simulink model "train_model"  (R2024b)
settings: Solver=VariableStepAuto  StartTime=0.0  StopTime=10.0  RelTol=1e-3
InitFcn:
  | m = 10000;
libraries: fuzblock x1
settings Model: Creator=Jan Tepel  LastModifiedBy=Jan Tepel

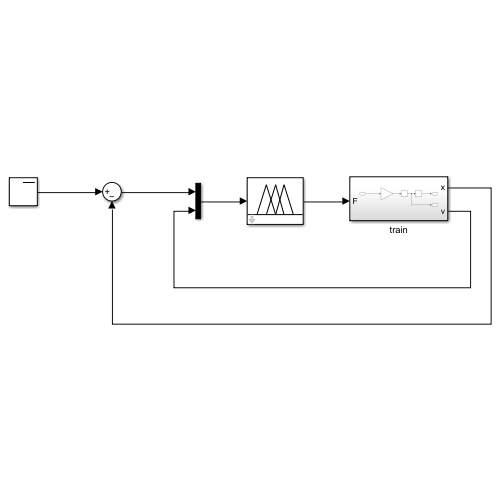
[thumbnail: Simulink's stored preview of the top-level diagram]
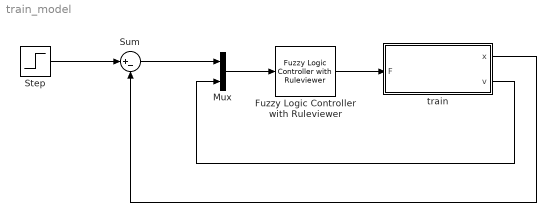
== system train_model ==
  Fuzzy Logic Controller with Ruleviewer : fuzblock/Fuzzy Logic  Controller  with Ruleviewer  fismatrix=fis  Ts=2
  Mux : Mux  Inputs=2
  Step : Step  SampleTime=0
  Sum : Sum  Inputs=|+-
  train : Subsystem
  wires:
  Step/1 -> Sum/1
  Sum/1 -> Mux/1
  train/2(v) -> Mux/2
  train/1(x) -> Sum/2
  Mux/1 -> Fuzzy Logic Controller with Ruleviewer/1
  Fuzzy Logic Controller with Ruleviewer/1 -> train/1(F)

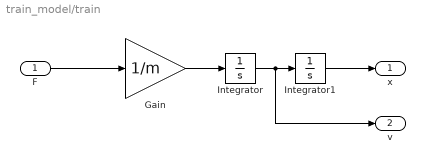
== system train_model/train ==
  F : Inport
  Gain : Gain  Gain=1/m
  Integrator : Integrator
  Integrator1 : Integrator
  x : Outport
  v : Outport  Port=2
  wires:
  F/1 -> Gain/1
  Gain/1 -> Integrator/1
  Integrator/1 -> v/1, Integrator1/1
  Integrator1/1 -> x/1
